simulink model "Middle_Ear_Filter"  (R2019b)
settings: Solver=VariableStepAuto  StartTime=0.0  StopTime=testtime  RelTol=1e-3
InitFcn:
  | Middle_Ear_Test_Parameters
StopFcn:
  | Verify_Middle_Ear
values from neighbouring files (symbols this model uses):
  Fs = 48e3    (= 48000)    [Middle_Ear_Test_Parameters.m]
  m11 = 1/(C^2+5.9761e+003*C+2.5255e+007)    [Middle_Ear_Test_Parameters.m]
  m12 = -2*C^2+2*2.5255e+007    [Middle_Ear_Test_Parameters.m]
  m13 = C^2-5.9761e+003*C+2.5255e+007    [Middle_Ear_Test_Parameters.m]
  m14 = C^2+5.6665e+003*C    [Middle_Ear_Test_Parameters.m]
  m15 = -2*C^2    [Middle_Ear_Test_Parameters.m]
  m16 = C^2-5.6665e+003*C    [Middle_Ear_Test_Parameters.m]
  m21 = 1/(C^2+6.4255e+003*C+1.3975e+008)    [Middle_Ear_Test_Parameters.m]
  m22 = -2*C^2+2*1.3975e+008    [Middle_Ear_Test_Parameters.m]
  m23 = C^2-6.4255e+003*C+1.3975e+008    [Middle_Ear_Test_Parameters.m]
  m24 = C^2+5.8934e+003*C+1.7926e+008    [Middle_Ear_Test_Parameters.m]
  m25 = -2*C^2+2*1.7926e+008    [Middle_Ear_Test_Parameters.m]
  m26 = C^2-5.8934e+003*C+1.7926e+008    [Middle_Ear_Test_Parameters.m]
  m31 = 1/(C^2+2.4891e+004*C+1.2700e+009)    [Middle_Ear_Test_Parameters.m]
  m32 = -2*C^2+2*1.2700e+009    [Middle_Ear_Test_Parameters.m]
  m33 = C^2-2.4891e+004*C+1.2700e+009    [Middle_Ear_Test_Parameters.m]
  m34 = (3.1137e+003*C+6.9768e+008)    [Middle_Ear_Test_Parameters.m]
  m35 = 2*6.9768e+008    (= 1395360000)    [Middle_Ear_Test_Parameters.m]
  m36 = -3.1137e+003*C+6.9768e+008    [Middle_Ear_Test_Parameters.m]
  megainmax = 2    [Middle_Ear_Test_Parameters.m]
undefined symbols (not defined in the file or in its folder): dfilt
libraries: dsparch4 x2, dspsrcs4 x2
settings Model: Creator=mblun  LastModifiedBy=t96f346
settings SFSimCC: CustomCodeUndefinedFunction=UseInterfaceOnly

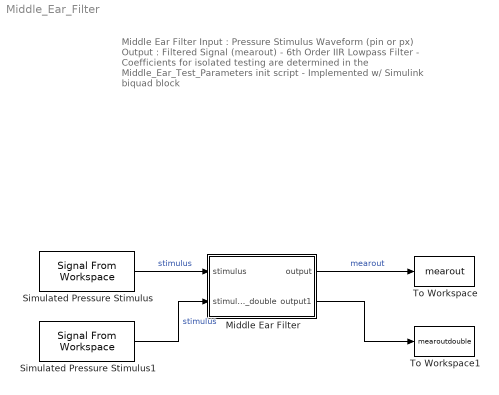
== system Middle_Ear_Filter ==
  note: Middle Ear Filter
      |
      | Input : Pressure Stimulus Waveform (pin or px)
      |
      | Output : Filtered Signal (mearout)
      |
      | - 6th Order IIR Lowpass Filter
      |
      | - Coefficients for isolated testing are determined in the Middle_Ear_Test_Parameters init script
      |
      | - Implemented w/ Simulink biquad block
  Middle Ear Filter : Subsystem
  Simulated Pressure Stimulus : dspsrcs4/Signal From Workspace  X=RxSignal  Ts=1/Fs  nsamps=1  OutputAfterFinalValue=Setting to zero  ignoreOrWarnInputAndFrameLengths=off  OutputFrames=off
  Simulated Pressure Stimulus1 : dspsrcs4/Signal From Workspace  X=RxSignalDouble  Ts=1/Fs  nsamps=1  OutputAfterFinalValue=Setting to zero  ignoreOrWarnInputAndFrameLengths=off  OutputFrames=off
  To Workspace : ToWorkspace  VariableName=mearout  SampleTime=-1
      settings: Save2DSignal=2-D array (concatenate along first dimension)
  To Workspace1 : ToWorkspace  VariableName=mearoutdouble  SampleTime=-1
      settings: Save2DSignal=2-D array (concatenate along first dimension)
  wires:
  Simulated Pressure Stimulus/1 -> Middle Ear Filter/1(stimulus)  "stimulus"
  Middle Ear Filter/1(output) -> To Workspace/1  "mearout"
  Simulated Pressure Stimulus1/1 -> Middle Ear Filter/2(stimulus_double)  "stimulus"
  Middle Ear Filter/2(output1) -> To Workspace1/1

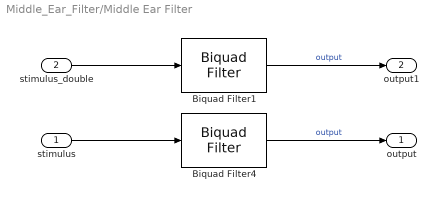
== system Middle_Ear_Filter/Middle Ear Filter ==
  stimulus : Inport
  stimulus_double : Inport  Port=2
  Biquad Filter1 : dsparch4/Biquad Filter  FilterSource=Dialog parameters  CoeffSource=Specify via dialog  FilterObject=dfilt.df2tsos([1 0.3 0.4],[1 0.1 0.2])  IIRFiltStruct=Direct form II transposed  BiQuadCoeffs=[m14*m11 m15*m11 m16*m11 1 m12*m11 m13*m11; m24*m21 m25*m21 m26*m21 1 m22*m21 m23*m21; m34*m31 m35*m31 m36*m31 1 m32*m31 m33*m31]  ScaleValues=[1 1 1 1/megainmax]  IC=0  ICnum=0  ICden=0  a0Flag=Warning  optimizeScaleValues=on  ScaleValueMode=Specify via input port (g)  roundingMode=Floor  overflowMode=on  scaleValueFracLength=14  denProdOutputFracLength=30  denAccumFracLength=30  secondMemoryFracLength=15
      settings: SourceProductName=DSP System Toolbox
  Biquad Filter4 : dsparch4/Biquad Filter  FilterSource=Dialog parameters  CoeffSource=Specify via dialog  FilterObject=dfilt.df2tsos([1 0.3 0.4],[1 0.1 0.2])  IIRFiltStruct=Direct form II transposed  BiQuadCoeffs=[m14*m11 m15*m11 m16*m11 1 m12*m11 m13*m11; m24*m21 m25*m21 m26*m21 1 m22*m21 m23*m21; m34*m31 m35*m31 m36*m31 1 m32*m31 m33*m31]  ScaleValues=[1 1 1 1/megainmax]  IC=0  ICnum=0  ICden=0  a0Flag=Warning  optimizeScaleValues=on  ScaleValueMode=Specify via input port (g)  roundingMode=Floor  overflowMode=on  scaleValueFracLength=14  denProdOutputFracLength=30  denAccumFracLength=30  secondMemoryFracLength=15
      settings: SourceProductName=DSP System Toolbox
  output : Outport  VectorParamsAs1DForOutWhenUnconnected=off
  output1 : Outport  Port=2  VectorParamsAs1DForOutWhenUnconnected=off
  wires:
  stimulus/1 -> Biquad Filter4/1
  Biquad Filter4/1 -> output/1  "output"
  Biquad Filter1/1 -> output1/1  "output"
  stimulus_double/1 -> Biquad Filter1/1
